simulink model "Quadcopter_ControllerWithNavigation"  (R2024a)
settings: Solver=FixedStepAuto  StartTime=0.0  StopTime=inf  RelTol=1e-3  EnableMultiTasking=on
undefined symbols (not defined in the file): SampleTime
libraries: slpidlib x10, px4uORBlib x7, simulink x4, px4lib x3, uavalgslib x3, simulink_extras x1, sharedutil x1, sharedtransform x1
(part 3 of 3)

== system Quadcopter_ControllerWithNavigation/Navigation/Quadcopter Navigation Algorithm/Read waypoint from QGroundControl Mission/Guidance Subsystem/Take-off/Ensure smooth ascend during Takeoff ==
  In1 : Inport
  Delay : Delay  DelayLength=1
  Gain : Gain  Gain=-1
  Gain1 : Gain  Gain=-1
  Rate : Constant  Value=0.01
  Relational Operator : RelationalOperator  Operator=<=  OutDataTypeStr=boolean  RndMeth=Simplest  InputSameDT=off
  Sum : Sum  Inputs=|++
  Switch : Switch  Criteria=u2 > Threshold  SaturateOnIntegerOverflow=off  InputSameDT=off
  Out1 : Outport
  wires:
  Rate/1 -> Sum/1
  Gain/1 -> Out1/1
  Relational Operator/1 -> Switch/2
  Switch/1 -> Gain/1
  In1/1 -> Gain1/1
  Sum/1 -> Relational Operator/2, Switch/3, Delay/1
  Gain1/1 -> Switch/1, Relational Operator/1
  Delay/1 -> Sum/2

== system Quadcopter_ControllerWithNavigation/Navigation/Quadcopter Navigation Algorithm/Read waypoint from QGroundControl Mission/Guidance Subsystem/Take-off/Maintain Current Yaw during TakeOff ==
  yaw_In : Inport
  Constant : Constant  Value=0
  Delay : Delay  DelayLength=1  InitialCondition=1
  Enabled Subsystem2 : Subsystem  TreatAsAtomicUnit=on
  yaw_Out : Outport
  wires:
  yaw_In/1 -> Enabled Subsystem2/1(yaw_In)
  Enabled Subsystem2/1(yaw_Out) -> yaw_Out/1
  Delay/1 -> Enabled Subsystem2/Enable
  Constant/1 -> Delay/1

== system Quadcopter_ControllerWithNavigation/Navigation/Quadcopter Navigation Algorithm/Read waypoint from QGroundControl Mission/Guidance Subsystem/Waypoint/Output signal conditioning ==
  Current Position : Inport
  LookAhead Point : Inport  Port=2
  Desired Yaw : Inport  Port=3
  Waypoint Type : Inport  Port=4
  Compare To Constant : simulink/Logic and Bit Operations/Compare To Constant  relop===  const=5  OutDataTypeStr=boolean
  Constant : Constant  Value=0  SampleTime=-1
  IsNaN : RelationalOperator  Operator=isNaN  OutDataTypeStr=boolean  RndMeth=Simplest  InputSameDT=off
  IsNaN1 : RelationalOperator  Operator=isNaN  OutDataTypeStr=boolean  RndMeth=Simplest  InputSameDT=off
  Matrix Concatenate1 : Concatenate  Mode=Multidimensional array  ConcatenateDimension=2
  OR : Logic  Operator=OR  IconShape=distinctive  AllPortsSameDT=off  OutDataTypeStr=boolean
  OR1 : Logic  Operator=OR  Inputs=1  IconShape=distinctive  AllPortsSameDT=off  OutDataTypeStr=boolean
  Reshape2 : Reshape  OutputDimensionality=Row vector (2-D)
  Reshape3 : Reshape  OutputDimensionality=Row vector (2-D)
  Switch : Switch  Criteria=u2 ~= 0  SaturateOnIntegerOverflow=off  InputSameDT=off
  Switch1 : Switch  Criteria=u2 > Threshold  SaturateOnIntegerOverflow=off  InputSameDT=off
  Transpose1 : Math  Operator=transpose
  xyzYaw : Outport
  wires:
  IsNaN1/1 -> OR1/1
  Reshape2/1 -> Matrix Concatenate1/2
  Matrix Concatenate1/1 -> Switch1/3
  OR/1 -> Switch1/2
  LookAhead Point/1 -> IsNaN1/1, Transpose1/1
  Compare To Constant/1 -> OR/2
  Transpose1/1 -> Matrix Concatenate1/1
  IsNaN/1 -> Switch/2
  Reshape3/1 -> Switch1/1
  Waypoint Type/1 -> Compare To Constant/1
  Switch1/1 -> xyzYaw/1
  Current Position/1 -> Reshape3/1
  OR1/1 -> OR/1
  Constant/1 -> Switch/1
  Switch/1 -> Reshape2/1
  Desired Yaw/1 -> Switch/3, IsNaN/1

== system Quadcopter_ControllerWithNavigation/Navigation/Quadcopter Navigation Algorithm/Path Correction from Onboard Computer/Guidance Subsystem/IDLE/Maintain Current Yaw during IDLE/Enabled Subsystem2 ==
  yaw_In : Inport
  Enable : EnablePort
  yaw_Out : Outport
  wires:
  yaw_In/1 -> yaw_Out/1

== system Quadcopter_ControllerWithNavigation/Navigation/Quadcopter Navigation Algorithm/Path Correction from Onboard Computer/Guidance Subsystem/Land/Ensure Smooth descend during Land/Enabled Subsystem ==
  In : Inport
  Enable : EnablePort
  Out : Outport
  wires:
  In/1 -> Out/1

== system Quadcopter_ControllerWithNavigation/Navigation/Quadcopter Navigation Algorithm/Path Correction from Onboard Computer/Guidance Subsystem/Land/Maintain Current Yaw during Land/Enabled Subsystem2 ==
  yaw_In : Inport
  Enable : EnablePort
  yaw_Out : Outport
  wires:
  yaw_In/1 -> yaw_Out/1

== system Quadcopter_ControllerWithNavigation/Navigation/Quadcopter Navigation Algorithm/Path Correction from Onboard Computer/Guidance Subsystem/Take-off/Maintain Current Yaw during TakeOff/Enabled Subsystem2 ==
  yaw_In : Inport
  Enable : EnablePort
  yaw_Out : Outport
  wires:
  yaw_In/1 -> yaw_Out/1

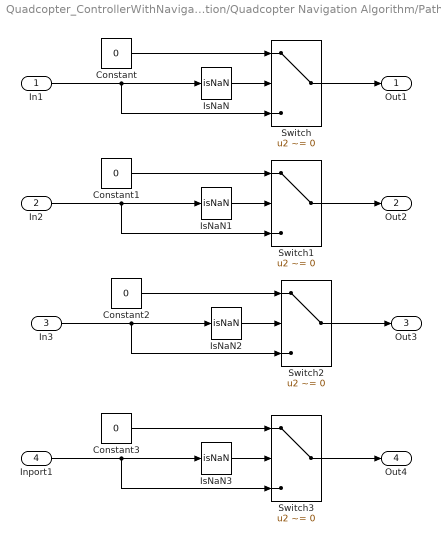
== system Quadcopter_ControllerWithNavigation/Navigation/Quadcopter Navigation Algorithm/Path Correction from Onboard Computer/Guidance Subsystem/Waypoint/Waypoints/NAN check ==
  In1 : Inport
  In2 : Inport  Port=2
  In3 : Inport  Port=3
  Inport1 : Inport  Port=4
  Constant{,1..3} (4 alike) : Constant  Value=0  SampleTime=-1
  IsNaN{,1..3} (4 alike) : RelationalOperator  Operator=isNaN  OutDataTypeStr=boolean  RndMeth=Simplest  InputSameDT=off
  Switch{,1..3} (4 alike) : Switch  Criteria=u2 ~= 0  SaturateOnIntegerOverflow=off  InputSameDT=off
  Out1 : Outport
  Out2 : Outport  Port=2
  Out3 : Outport  Port=3
  Out4 : Outport  Port=4
  wires:
  Switch/1 -> Out1/1
  In1/1 -> Switch/3, IsNaN/1
  Constant/1 -> Switch/1
  IsNaN/1 -> Switch/2
  Switch1/1 -> Out2/1
  IsNaN1/1 -> Switch1/2
  In2/1 -> Switch1/3, IsNaN1/1
  Constant1/1 -> Switch1/1
  Switch2/1 -> Out3/1
  IsNaN2/1 -> Switch2/2
  In3/1 -> Switch2/3, IsNaN2/1
  Constant2/1 -> Switch2/1
  Inport1/1 -> Switch3/3, IsNaN3/1
  Switch3/1 -> Out4/1
  Constant3/1 -> Switch3/1
  IsNaN3/1 -> Switch3/2

== system Quadcopter_ControllerWithNavigation/Navigation/Quadcopter Navigation Algorithm/Read waypoint from QGroundControl Mission/Guidance Subsystem/IDLE/Maintain Current Yaw during IDLE/Enabled Subsystem2 ==
  yaw_In : Inport
  Enable : EnablePort
  yaw_Out : Outport
  wires:
  yaw_In/1 -> yaw_Out/1

== system Quadcopter_ControllerWithNavigation/Navigation/Quadcopter Navigation Algorithm/Read waypoint from QGroundControl Mission/Guidance Subsystem/Land/Ensure Smooth descend during Land/Enabled Subsystem ==
  In : Inport
  Enable : EnablePort
  Out : Outport
  wires:
  In/1 -> Out/1

== system Quadcopter_ControllerWithNavigation/Navigation/Quadcopter Navigation Algorithm/Read waypoint from QGroundControl Mission/Guidance Subsystem/Land/Maintain Current Yaw during Land/Enabled Subsystem2 ==
  yaw_In : Inport
  Enable : EnablePort
  yaw_Out : Outport
  wires:
  yaw_In/1 -> yaw_Out/1

== system Quadcopter_ControllerWithNavigation/Navigation/Quadcopter Navigation Algorithm/Read waypoint from QGroundControl Mission/Guidance Subsystem/Take-off/Maintain Current Yaw during TakeOff/Enabled Subsystem2 ==
  yaw_In : Inport
  Enable : EnablePort
  yaw_Out : Outport
  wires:
  yaw_In/1 -> yaw_Out/1
